simulink model "Valvula"  (Simulink 10.3)
settings: Solver=ode3  StartTime=0.0  StopTime=1000  RelTol=1e-3  EnableMultiTasking=on
undefined symbols (not defined in the file or in its folder): Fh0
settings Model: Creator=Marcelo  LastModifiedBy=Fer
settings SolverCC: ShapePreserveControl=EnableAll
settings DataIOCC: SaveOutput=off  SaveTime=off
settings OptimizationCC: BooleanDataType=off
settings DebuggingCC: SaveWithParameterizedLinksMsg=none  SignalResolutionControl=TryResolveAllWithWarning  MultiTaskDSMMsg=warning  MultiTaskCondExecSysMsg=none
settings HardwareCC: TargetUnknown=on

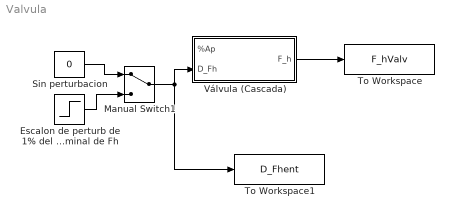
== system Valvula ==
  Escalon de perturb de 1% del valor nominal de Fh : Step  Time=50  Before=Fh0  After=Fh0*1.01  SampleTime=0
  Manual Switch1 : ManualSwitch
  Sin perturbacion : Constant  Value=0
  To Workspace : ToWorkspace  VariableName=F_hValv  SampleTime=-1
  To Workspace1 : ToWorkspace  VariableName=D_Fhent  SampleTime=-1
  Válvula (Cascada) : Subsystem
  wires:
  Manual Switch1/1 -> To Workspace1/1, Válvula (Cascada)/2(D_Fh)
  Sin perturbacion/1 -> Manual Switch1/1
  Escalon de perturb de 1% del valor nominal de Fh/1 -> Manual Switch1/2
  Válvula (Cascada)/1(F_h) -> To Workspace/1

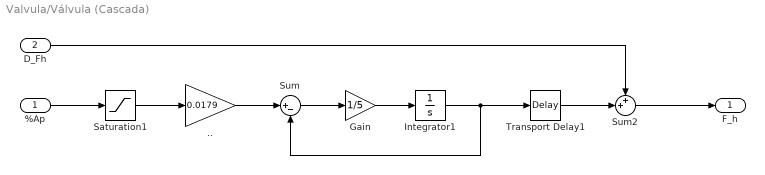
== system Valvula/Válvula (Cascada) ==
  %Ap : Inport
  D_Fh : Inport  Port=2
  .. : Gain  Gain=0.0179
  Gain : Gain  Gain=1/5
  Integrator1 : Integrator  InitialCondition=Fh0
  Saturation1 : Saturate  UpperLimit=100  LowerLimit=0
  Sum : Sum  Inputs=|+-
  Sum2 : Sum  Inputs=++|
  Transport Delay1 : TransportDelay  InitialOutput=Fh0
  F_h : Outport
  wires:
  D_Fh/1 -> Sum2/1
  Sum2/1 -> F_h/1
  %Ap/1 -> Saturation1/1
  Saturation1/1 -> ../1
  Sum/1 -> Gain/1
  Gain/1 -> Integrator1/1
  Integrator1/1 -> Transport Delay1/1, Sum/2
  ../1 -> Sum/1
  Transport Delay1/1 -> Sum2/2
